simulink model "elec_mosfet"  (R2014a)
settings: Solver=ode15s  StartTime=0.0  StopTime=t_sim  RelTol=1e-3
PreLoadFcn:
  | Vg = 5;
  | Vds_min = 0;
  | Vds_max = 4;
  | t_sim = 1;
libraries: fl_lib x4, nesl_utility x3, elec_lib x1, simulink x1
Description:
  | MOSFET Characteristics
  | 
  | This example shows generation of the characteristic curves for an
  | N-channel MOSFET. Define the vector of gate voltages and minimum
  | and maximum drain-source voltages by double clicking on the block
  | labeled 'Define Vg and Vds'. Then double click on the block labeled
  | 'Generate Characteristics'.
  | 
  | This type of plot can be compared against a manufacturer
  | datasheet to confirm a correct implementation of the MOSFET
  | parameters. You can also use this model to examine the MOSFET
  | characteristics in the reverse region by specifying a range of
  | negative Vds values.
  | 
  | To explore the properties of a P-channel MOSFET, copy a
  | P-Channel MOSFET from the library to replace the N-channel
  | device, taking care to swap over the two output connections so
  | that the source is still connected to ground. To specify normal
  | operation, the vector of gate voltages should be negative, and
  | the Vds range of values should be negative.
  | 
  | 
  | 
  | Copyright 2008-2014 The MathWorks, Inc.
settings Model: ExtModeAutoUpdateStatusClock=off  Creator=MathWorks  LastModifiedBy=User
settings DataIOCC: SignalLoggingSaveFormat=ModelDataLogs  OutputOption=SpecifiedOutputTimes  OutputTimes=[0:t_sim/100:t_sim]  Refine=5
settings OptimizationCC: ExpressionDepthLimit=2147483647  InitFltsAndDblsToZero=on  EfficientMapNaN2IntZero=off
settings DebuggingCC: SaveWithParameterizedLinksMsg=none  UnderspecifiedInitializationDetection=Classic  SignalResolutionControl=TryResolveAllWithWarning  SolverPrmCheckMsg=none  FcnCallInpInsideContextMsg=UseLocalSettings  StateNameClashWarn=warning
settings GRTTargetCC: TargetFcnLib=ansi_tfl_tmw.mat  CombineOutputUpdateFcns=off  GRTInterface=on

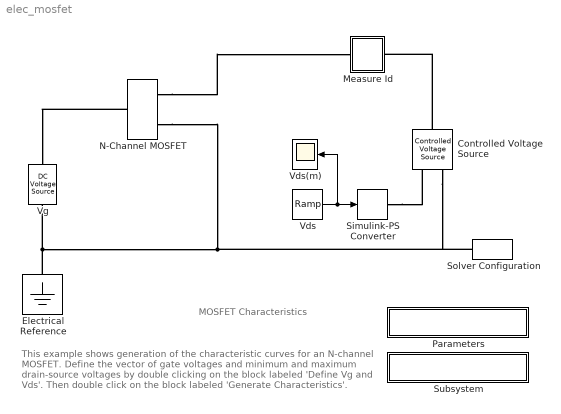
== system elec_mosfet ==
  note: MOSFET Characteristics
  note: This example shows generation of the characteristic curves for an
      | N-channel MOSFET. Define the vector of gate voltages and minimum
      | and maximum drain-source voltages by double clicking on the block
      | labeled 'Define Vg and Vds'. Then double click on the block labeled
      | 'Generate Characteristics'.
  Controlled Voltage Source : fl_lib/Electrical/Electrical Sources/Controlled Voltage Source
  Electrical Reference : fl_lib/Electrical/Electrical Elements/Electrical Reference
  Measure Id : Subsystem
  N-Channel MOSFET : elec_lib/Semiconductor Devices/N-Channel MOSFET  parameterization=2  prmDatasheet=1  prmEquCoeff=1  Beta=5 A/V^2  Rds=0.025 Ohm  Id=6 A  Vgs=10 V  Vth=1.7 V  lam=0 1/V  Tmeas=25 C  RS=0.001 Ohm  RD=0.001 Ohm  C_param=1  C_GS=270 pF  C_GD=80 pF  C_iss=350 pF  C_rss=80 pF  C_oss=0 pF  charge_linearity_param=1  C_OX=200 pF  V_C_OX=-0.5 V  dVth_dT=-6 mV/K  Rds_T2=0.037 Ohm  Tmeas2=125 C  BEXDatasheet=-1.5  BEXEquCoeff=-1.5  TdeviceDatasheet=25 C  TdeviceEquCoeff=25 C  Rth=[ 0 10 ] K/W  thermal_mass_parameterization=1  thermal_mass=[ 0 1 ] J/K  thermal_time_constant=[ 0 10 ] s  thermal_mass_initial_temperatures=[ 25 25 ] C
  Parameters : Subsystem  mask(MOSFET Test Parameters){Vg_vec=[3 3.5 4 4.5 5 6 10], Vds_min=0, Vds_max=4}
      mask prompts: Vg_vec "Vector of gate voltages Vg"; Vds_min "Minimum drain-source voltage"; Vds_max "Maximum drain-source voltage"
      mask help: Define a range of base currents and collector-emitter voltages over which to plot collector current
      mask Display: disp('Define Vg and Vds')
  Simulink-PS Converter : nesl_utility/Simulink-PS Converter  PhysicalDomain=network_engine_domain  SubClassName=ps_input  LeftPortType=input  RightPortType=output  PseudoPeriodic=off  Frequencies=[]  NoiseDistribution=none  NoiseParameters=[]  Unit=1  AffineConversion=off  InputFiltering=off  SimscapeFilterOrder=1  InputFilterTimeConstant=.001  UdotUserProvided=0
  Solver Configuration : nesl_utility/Solver Configuration  PhysicalDomain=network_engine_domain  SubClassName=solver  LeftPortType=input  RightPortType=generic  Accelerate=off  Tones=[]  Harmonics=[]  SimulateNoise=off  Profile=off  UseLocalSampling=off  EnableSwitchedLinearOptims=on  FrequencyDomain=off  UseCCode=off  RelTol=0.001  AbsTol=1e-06  MinStep=1e-09  ToWorkspace=off  DoDC=on  ResidualTolerance=1e-9  UseLocalSolver=off  LocalSolverChoice=NE_BACKWARD_EULER_ADVANCER  LocalSolverSampleTime=.001  DoFixedCost=off  MaxNonlinIter=3  MaxModeIter=2  LinearAlgebra=Sparse  DelaysMemoryBudget=1024  AutomaticFiltering=on  FilteringTimeConstant=0.001
  Subsystem : Subsystem
      settings: OpenFcn=elec_mosfet_callback
      mask Display: disp('Generate Characteristics')
  Vds : simulink/Sources/Ramp  slope=(Vds_max-Vds_min)/t_sim  start=0  X0=Vds_min
  Vds(m) : Scope
      settings: TimeRange=1  YMin=0  YMax=4  SaveName=Vds
  Vg : fl_lib/Electrical/Electrical Sources/DC Voltage Source  v0=Vg V
  wires:
  Vds/1 -> Simulink-PS Converter/1, Vds(m)/1
  connections:
  Electrical Reference/LConn1 -- Solver Configuration/RConn1 -- Controlled Voltage Source/RConn2 -- N-Channel MOSFET/RConn2 -- Vg/RConn1
  N-Channel MOSFET/LConn1 -- Vg/LConn1
  N-Channel MOSFET/RConn1 -- Measure Id/RConn1
  Controlled Voltage Source/LConn1 -- Measure Id/LConn1
  Simulink-PS Converter/RConn1 -- Controlled Voltage Source/RConn1

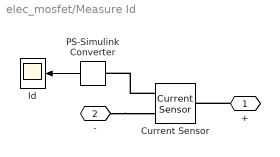
== system elec_mosfet/Measure Id ==
  Current Sensor : fl_lib/Electrical/Electrical Sensors/Current Sensor
  Id : Scope
      settings: TimeRange=1  YMin=0  YMax=30  SaveName=Id
  PS-Simulink Converter : nesl_utility/PS-Simulink Converter  PhysicalDomain=network_engine_domain  SubClassName=ps_output  LeftPortType=input  RightPortType=output  PseudoPeriodic=off  Frequencies=[]  Unit=1  AffineConversion=off
  + : PMIOPort  Port=1  Side=Left
  - : PMIOPort  Port=2  Side=Right
  wires:
  PS-Simulink Converter/1 -> Id/1
  connections:
  +/RConn1 -- Current Sensor/LConn1
  -/RConn1 -- Current Sensor/RConn2
  Current Sensor/RConn1 -- PS-Simulink Converter/LConn1

== system elec_mosfet/Parameters ==

== system elec_mosfet/Subsystem ==
